simulink model "sim_Motor_2kW_openloop_delay"  (Simulink 7.9)
settings: Solver=ode23  StartTime=0.0  StopTime=0.01  RelTol=1e-3
libraries: powerlib x18
settings Model: Creator=Kun Zhang  LastModifiedBy=LYN
settings SolverCC: AutoInsertRateTranBlk=on
settings GRTTargetCC: CombineOutputUpdateFcns=off  GRTInterface=on

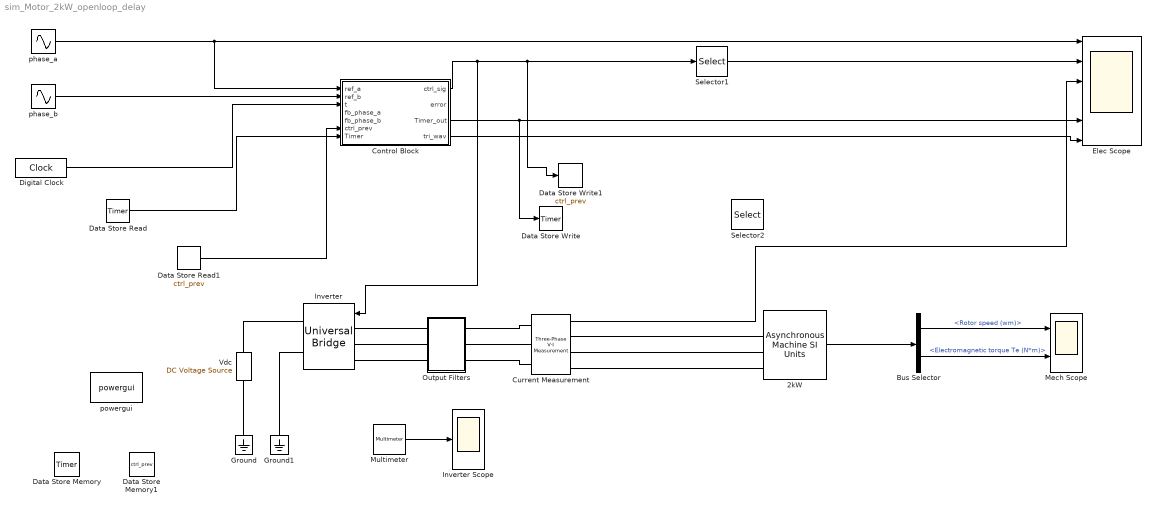
== system sim_Motor_2kW_openloop_delay ==
  2kW : powerlib/Machines/Asynchronous Machine SI Units  PresetModel=No  MechanicalLoad=Torque Tm  ShowDetailedParameters=on  RotorType=Squirrel-cage  ReferenceFrame=Rotor  NominalParameters=[ 2000, 220, 50 ]  Stator=[ 1.115 0.005974]  Rotor=[ 1.083 0.005974]  Cage1=[ 0.022 0.226/377]  Cage2=[ 0.022 0.226/377]  Lm=0.2037  Mechanical=[0.02 0.005752 2]  PolePairs=2  InitialConditions=[1 0 0 0 0 0 0 0]  Units=SI  LoadFlowParameters=1492000  SimulateSaturation=off  Saturation=[14.03593122, 27.81365428, 53.79336849, 72.68890987, 97.98006896, 148.6815601, 215.7428561, 302.9841135, 428.7778367 ; 230, 322, 414, 460, 506, 552, 598, 644, 690]  TsPowergui=0  TsBlock=-1  IterativeModel=Forward Euler  Pmec=0
  Bus Selector : BusSelector  OutputSignals=Mechanical.Rotor speed (wm),Mechanical.Electromagnetic torque Te (N*m)
  Control Block : MATLAB Function  TreatAsAtomicUnit=on
  Current Measurement : powerlib/Measurements/Three-Phase V-I Measurement  VoltageMeasurement=no  SetLabelV=off  LabelV=Vabc  Vpu=off  VpuLL=off  CurrentMeasurement=yes  SetLabelI=off  LabelI=Iabc  Ipu=off  Pbase=100e6  Vbase=500e3  OutputType=Complex  PhasorSimulation=off  PSBequivalent=0
  Data Store Memory : DataStoreMemory  DataStoreName=Timer  ReadBeforeWriteMsg=warning  WriteAfterWriteMsg=warning  WriteAfterReadMsg=warning  InitialValue=[0 0 0]
  Data Store Memory1 : DataStoreMemory  DataStoreName=ctrl_prev  ReadBeforeWriteMsg=warning  WriteAfterWriteMsg=warning  WriteAfterReadMsg=warning  InitialValue=[0 0 0 0 0 0]
  Data Store Read : DataStoreRead  DataStoreName=Timer
  Data Store Read1 : DataStoreRead  DataStoreName=ctrl_prev  DataStoreElements=ctrl_prev
  Data Store Write : DataStoreWrite  DataStoreName=Timer
  Data Store Write1 : DataStoreWrite  DataStoreName=ctrl_prev
  Digital Clock : DigitalClock  SampleTime=1e-7
  "Elec Scope " : Scope  NumInputPorts=6
      settings: TimeRange=0.00016  YMin=0.29~0~-1.5e-15~-1~0~-1.25  YMax=0.38~1~7.5e-16~1~30~1.25  SaveName=motor_2kW_elec
  Ground : powerlib/Elements/Ground  LConnTagsString=a
  Ground1 : powerlib/Elements/Ground  LConnTagsString=a
  Inverter : powerlib/Power Electronics/Universal Bridge  Arms=3  SnubberResistance=5000  SnubberCapacitance=inf  Device=IGBT / Diodes  Ron=1e-3  Lon=0  ForwardVoltages="[  0  0  ]"  ForwardVoltage=0  GTOparameters=[ 10e-6 , 20e-6 ]  IGBTparameters=[ 1e-6 , 1e-6]  Measurements=Device voltages  Measurements_2=None  converterType=Rectifier
  Inverter Scope : Scope
      settings: TimeRange=5e-05  YMin=0  YMax=400  SaveName=motor_2kW_Inverter
  Mech Scope : Scope  NumInputPorts=2
      settings: TimeRange=0.01  YMin=-1.2e-25~-1.3e-22  YMax=0~-1.17549e-38  SaveName=motor_2kW_mech
  Multimeter : powerlib/Measurements/Multimeter  PhasorSimulation=off  OutputType=Complex  sel=[1 2 3 4]  L=6  Gain=[1 1 1 1]  yselected={'Usw1: Inverter','Usw2: Inverter','Usw3: Inverter','Usw4: Inverter'};  PSBOutputType=1  PSBequivalent=0  AxesSetting=[0,0.1,-100,100]  Display=1  SavedBlockNames=-11
  Output Filters : Subsystem
  Selector1 : Selector  InputPortWidth=6  IndexOptions=Index vector (dialog)  Indices=[1 2]  OutputSizes=1
  Selector2 : Selector  InputPortWidth=3  IndexOptions=Index vector (dialog)  Indices=[1]  OutputSizes=1
  Vdc : powerlib/Electrical Sources/DC Voltage Source  Amplitude=400  Measurements=None
  "phase_a " : Sin  Frequency=2*pi*300  SampleTime=0.1e-6
  "phase_b " : Sin  Frequency=2*pi*300  Phase=2*pi/3  SampleTime=0.1e-6
  powergui : powerlib/powergui  Priority=1  SimulationMode=Discrete  SolverType=Tustin  SampleTime=1e-7  frequency=60  SPID=off  DisableSnubberDevices=off  DisableRonSwitches=off  DisableVfSwitches=off  SwTol=0  Interpol=off  DisplayEquations=off  FunctionMessages=off  frequencyindice=50  Pbase=100e6  ErrMax=1e-4  Iterations=50  UnitsV=kV  UnitsW=MW  echomessages=off  HookPort=off  EnableUseOfTLC=off  x0status=blocks  RestoreLinks=warning  ResistiveCurrentMeasurement=off  Ylog=off  Xlog=on  ShowGrid=off  save=off  variable=ZData  structure=motor_2kW_  ZoomFFT=off  StartTime=0.0  cycles=1  DisplayStyle=1  fundamental=60  FreqAxis=off  MaxFrequency=1000  frequencyindicesteady=1  display=off  methode=off
  wires:
  2kW/1 -> Bus Selector/1
  Bus Selector/1 -> Mech Scope/1  "<Rotor speed (wm)>"
  Bus Selector/2 -> Mech Scope/2  "<Electromagnetic torque Te (N*m)>"
  "phase_b "/1 -> Control Block/2(ref_b)
  Control Block/1(ctrl_sig) -> Inverter/1, Selector1/1, Data Store Write1/1
  Digital Clock/1 -> Control Block/3(t)
  "phase_a "/1 -> Control Block/1(ref_a), "Elec Scope "/1
  Multimeter/1 -> Inverter Scope/1
  Data Store Read/1 -> Control Block/7(Timer)
  Control Block/4(tri_wav) -> "Elec Scope "/6
  Control Block/3(Timer_out) -> "Elec Scope "/5, Data Store Write/1
  Data Store Read1/1 -> Control Block/6(ctrl_prev)
  Selector1/1 -> "Elec Scope "/2
  Current Measurement/1 -> "Elec Scope "/3
  connections:
  Ground/LConn1 -- Vdc/LConn1
  Vdc/RConn1 -- Inverter/RConn1
  Inverter/RConn2 -- Ground1/LConn1
  Inverter/LConn1 -- Output Filters/LConn1
  Output Filters/LConn2 -- Inverter/LConn2
  Inverter/LConn3 -- Output Filters/LConn3
  Output Filters/RConn1 -- Current Measurement/LConn1
  Output Filters/RConn2 -- Current Measurement/LConn2
  Output Filters/RConn3 -- Current Measurement/LConn3
  Current Measurement/RConn3 -- 2kW/LConn3
  Current Measurement/RConn2 -- 2kW/LConn2
  Current Measurement/RConn1 -- 2kW/LConn1

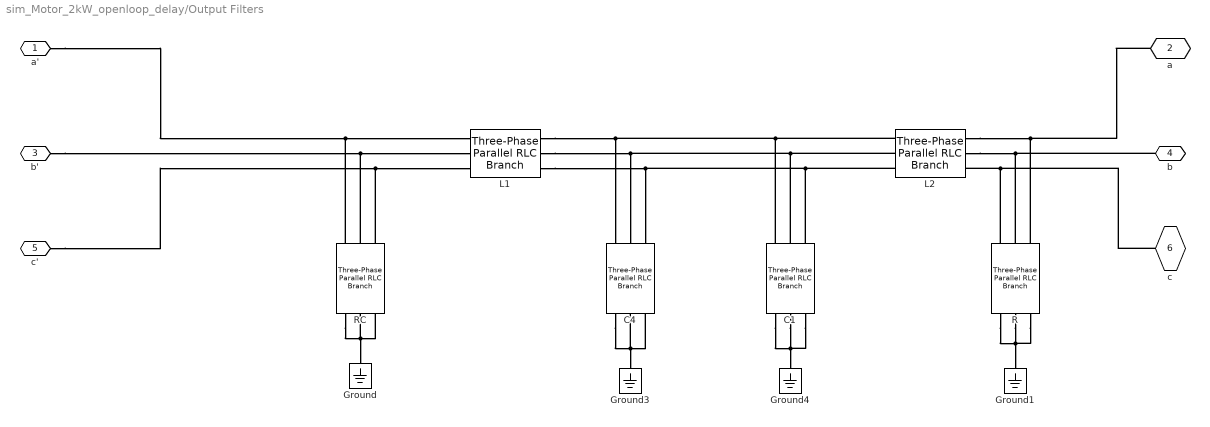
== system sim_Motor_2kW_openloop_delay/Output Filters ==
  C1 : powerlib/Elements/Three-Phase Parallel RLC Branch  LConnTagsString=A|B|C  RConnTagsString=A|B|C  BranchType=C  Resistance=1.5e6  Inductance=0.15e-5  Capacitance=10e-9  Measurements=None
  C4 : powerlib/Elements/Three-Phase Parallel RLC Branch  LConnTagsString=A|B|C  RConnTagsString=A|B|C  BranchType=C  Resistance=1.5e6  Inductance=0.15e-5  Capacitance=22e-6  Measurements=None
  Ground{,1,3..4} (4 alike) : powerlib/Elements/Ground  LConnTagsString=a
  L1 : powerlib/Elements/Three-Phase Parallel RLC Branch  LConnTagsString=A|B|C  RConnTagsString=A|B|C  BranchType=L  Resistance=1  Inductance=0.7e-1  Capacitance=1e-6  Measurements=None
  L2 : powerlib/Elements/Three-Phase Parallel RLC Branch  LConnTagsString=A|B|C  RConnTagsString=A|B|C  BranchType=L  Resistance=1  Inductance=1.4e-3  Capacitance=1e-6  Measurements=None
  "R " : powerlib/Elements/Three-Phase Parallel RLC Branch  LConnTagsString=A|B|C  RConnTagsString=A|B|C  BranchType=R  Resistance=100  Inductance=0.15e-5  Capacitance=20e-9  Measurements=None
  RC : powerlib/Elements/Three-Phase Parallel RLC Branch  LConnTagsString=A|B|C  RConnTagsString=A|B|C  BranchType=RC  Resistance=1.5e6  Inductance=0.15e-5  Capacitance=22e-6  Measurements=None
  " a'" : PMIOPort  Port=1  Side=Left
  a : PMIOPort  Port=2  Side=Right
  b' : PMIOPort  Port=3  Side=Left
  b : PMIOPort  Port=4  Side=Right
  c' : PMIOPort  Port=5  Side=Left
  c : PMIOPort  Port=6  Side=Right
  connections:
  RC/RConn1 -- " a'"/RConn1 -- L1/LConn1
  RC/RConn2 -- b'/RConn1 -- L1/LConn2
  RC/RConn3 -- c'/RConn1 -- L1/LConn3
  RC/LConn3 -- RC/LConn1 -- Ground/LConn1 -- RC/LConn2
  "R "/RConn2 -- L2/RConn2 -- b/RConn1
  "R "/LConn1 -- "R "/LConn3 -- "R "/LConn2 -- Ground1/LConn1
  L1/RConn1 -- L2/LConn1 -- C1/RConn1 -- C4/RConn1
  L1/RConn2 -- C1/RConn2 -- L2/LConn2 -- C4/RConn2
  L1/RConn3 -- C1/RConn3 -- L2/LConn3 -- C4/RConn3
  a/RConn1 -- L2/RConn1 -- "R "/RConn3
  c/RConn1 -- "R "/RConn1 -- L2/RConn3
  C4/LConn2 -- Ground3/LConn1 -- C4/LConn1 -- C4/LConn3
  C1/LConn3 -- C1/LConn1 -- Ground4/LConn1 -- C1/LConn2

== matlab function Control Block ==
  data: ref_a input double; ctrl_sig output double; ref_b input double; t input double; error output double; fb_phase_a input double; fb_phase_b input double; ctrl_prev input double; Timer input double; Timer_out output double; tri_wav output double
function    [ctrl_sig,error,Timer_out,tri_wav]= ctrl_blk(ref_a,ref_b,t,fb_phase_a,fb_phase_b,ctrl_prev,Timer)
%%%%%%%%%%%%%%%%%%%%%%%%%%%%%%%%%%%%%%%%%%%%%%%%%%%%%%%%%%%%%%%%%%%%%%%%%%%%%%%%%%%%%%%%%%%%%%%%%%%%%%%%%%%%%%%%%%%%%%%%%%%%%%%%%%%%%%%%%%%%%%%%%%%%%%%%%%%%%%%%%
%                                                                                                                                                               %
%           The aim is to:                                                                                                                                      %
%           generate 3-phase PWM waveform using principle of PWM in simulink                                                                                    %
%           Version 1, written by Kun Zhang                                                                                                                     %
%                                                                                                                                                               %
%           The input parameters are                                                                                                                            %
%           phase_a: reference signal a                                                                                                                         %
%           phase_b: reference signal b                                                                                                                         %
%           t: running time                                                                                                                                     %
%           fb_phase_a: feedback signal a                                                                                                                       %
%           fb_phase_a: feedback signal b                                                                                                                       %
%                                                                                                                                                               %
%%%%%%%%%%%%%%%%%%%%%%%%%%%%%%%%%%%%%%%%%%%%%%%%%%%%%%%%%%%%%%%%%%%%%%%%%%%%%%%%%%%%%%%%%%%%%%%%%%%%%%%%%%%%%%%%%%%%%%%%%%%%%%%%%%%%%%%%%%%%%%%%%%%%%%%%%%%%%%%%%
%space reserved for gloabal variables declaration


%%%%%%%%%%%%%%%%%%%%%%%%%%%%%%%%%%%%%%%%%%%%%%%%%%%%%%%%%%%%%%%%%%%%%%%%%%%%%%%%%%%%%%%%%%%%%%%%%%%%%%%%%%%%%%%%%%%%%%%%%%%%%%%%%%%%%%%%%%%%%%%%%%%%%%%%%%%%%%%%%
%Parameter settings
REF_AMP= 1;                         %magnitude of reference
REF_FREQ= 300;                      %frequency of reference
AMP_MOD= 0.9;                       %amplitude modulation ratio=M(control)/M(tri)
FREQ_MOD= 50;                       %frequency modulation ratio=f(tri)/f(control)

TRI_AMP= REF_AMP/AMP_MOD;           %triangluar amplitude
TRI_FREQ= FREQ_MOD*REF_FREQ;        %triangular frequency
TRI_PER= 1/TRI_FREQ;                %triangular period

%SAMP_FREQ= 10*1000000;              %sampling frequency
%SAMP_PER= 1/SAMP_FREQ;              %sampling period


%%%%%%%%%%%%%%%%%%%%%%%%%%%%%%%%%%%%%%%%%%%%%%%%%%%%%%%%%%%%%%%%%%%%%%%%%%%%%%%%%%%%%%%%%%%%%%%%%%%%%%%%%%%%%%%%%%%%%%%%%%%%%%%%%%%%%%%%%%%%%%%%%%%%%%%%%%%%%%%%%
ref_c= -ref_a-ref_b;                                                            %phase_c obatined by phase_a and phase_b
tri_wav= (2*TRI_AMP/(TRI_PER/2))*abs(mod(t,TRI_PER)-TRI_PER/2)-TRI_AMP;         %triangular wave 

%Leg 1
if      ref_a>tri_wav;              
        if      ctrl_prev(2)==REF_AMP                                           %if it is a falling edge for switch 2
                pwm_1= 0;               pwm_2= 0;                               %if yes, hold pwm_1   
                Timer(1)= 1;                                                    %Timer1 is 1 indicates the onset of delay                                                     
        end
        if      Timer(1)>0&&Timer(1)<30                                         %Time1<30*1e-07=3us dalay period     
                pwm_1= 0;               pwm_2= 0;                               %if yes, hold pwm_1, increment Timer 1          
                Timer(1)= Timer(1)+1; 
        else    pwm_1= REF_AMP;         pwm_2= 0;                               %if Time==0(not an edge) or Timer>=21(beyond delay period)
                Timer(1)= 0;                                                    %set Timer to 0
        end
else                                                                            %if ref_a<tri_wav; 
        if      ctrl_prev(1)==REF_AMP                                           %if it is a falling edge for switch 1
                pwm_1=0;                pwm_2= 0;                               %if yes, hold pwm_2  
                Timer(1)= 1;                                                    %Timer1 = 1 indicates the onset of delay
        end
        if      Timer(1)>0&&Timer(1)<30                                         %Time1<22*1e-07=2.2us dalay period     
                pwm_1=0;          pwm_2= 0;                                     %if yes, hold pwm_1, increment Timer 1          
                Timer(1)= Timer(1)+1; 
        else    pwm_1=0;                pwm_2= REF_AMP;                               
        end           
end

%Leg 2
if      ref_a>tri_wav;              
        if      ctrl_prev(4)==REF_AMP                                           %if it is a falling edge for switch 2
                pwm_3= 0;               pwm_4= 0;                               %if yes, hold pwm_1   
                Timer(2)= 1;                                                    %Timer1 is 1 indicates the onset of delay                                                     
        end
        if      Timer(2)>0&&Timer(2)<30                                         %Time1<22*1e-07=2.2us dalay period     
                pwm_3= 0;               pwm_4= 0;                               %if yes, hold pwm_1, increment Timer 1          
                Timer(2)= Timer(2)+1; 
        else    pwm_3= REF_AMP;         pwm_4= 0;                               %if Time==0(not an edge) or Timer>=21(beyond delay period)
                Timer(2)= 0;                                                    %set Timer to 0
        end
else                                                                            %if ref_a<tri_wav; 
        if      ctrl_prev(3)==REF_AMP                                           %if it is a falling edge for switch 1
                pwm_3=0;                pwm_4= 0;                               %if yes, hold pwm_2  
                Timer(2)= 1;                                                    %Timer1 = 1 indicates the onset of delay
        end
        if      Timer(2)>0&&Timer(2)<30                                      	%Time1<22*1e-07=2.2us dalay period     
                pwm_3=0;          pwm_4= 0;                                     %if yes, hold pwm_1, increment Timer 1          
                Timer(2)= Timer(2)+1; 
        else    pwm_3=0;                pwm_4= REF_AMP;                               
        end           
end

%Leg 3
if      ref_a>tri_wav;              
        if      ctrl_prev(6)==REF_AMP                                           %if it is a falling edge for switch 2
                pwm_5= 0;               pwm_6= 0;                               %if yes, hold pwm_1   
                Timer(3)= 1;                                                    %Timer1 is 1 indicates the onset of delay                                                     
        end
        if      Timer(3)>0&&Timer(3)<30                                         %Time1<22*1e-07=2.2us dalay period     
                pwm_5= 0;               pwm_6= 0;                               %if yes, hold pwm_1, increment Timer 1          
                Timer(3)= Timer(3)+1; 
        else    pwm_5= REF_AMP;         pwm_6= 0;                               %if Time==0(not an edge) or Timer>=21(beyond delay period)
                Timer(3)= 0;                                                    %set Timer to 0
        end
else                                                                            %if ref_a<tri_wav; 
        if      ctrl_prev(5)==REF_AMP                                           %if it is a falling edge for switch 1
                pwm_5=0;                pwm_6= 0;                               %if yes, hold pwm_2  
                Timer(3)= 1;                                                    %Timer1 = 1 indicates the onset of delay
        end
        if      Timer(3)>0&&Timer(3)<30                                     	%Time1<22*1e-07=2.2us dalay period     
                pwm_5=0;          pwm_6= 0;                                     %if yes, hold pwm_1, increment Timer 1          
                Timer(3)= Timer(3)+1; 
        else    pwm_5=0;                pwm_6= REF_AMP;                               
        end           
end


%%%%%%%%%%%%%%%%%%%%%%%%%%%%%%%%%%%%%%%%%%%%%%%%%%%%%%%%%%%%%%%%%%%%%%%%%%%%%%%%%%%%%%%%%%%%%%%%%%%%%%%%%%%%%%%%%%%%%%%%%%%%%%%%%%%%%%%%%%%%%%%%%%%%%%%%%%%%%%%%%
ctrl_sig= [pwm_1 pwm_2 pwm_3 pwm_4 pwm_5 pwm_6];        %PWM output
mag_fb= 200;                                            %magnitude of feedback
error= fb_phase_a-mag_fb*ref_a;                         %error
Timer_out= Timer;
